simulink model "test_pkt_reorder"  (Simulink 6.2)
settings: Solver=ode45  StartTime=0.0  StopTime=200000  RelTol=1e-3
libraries: xbsIndex_r3 x556, casper_library x22, xps_library x21, simulink x1
(part 2 of 3)

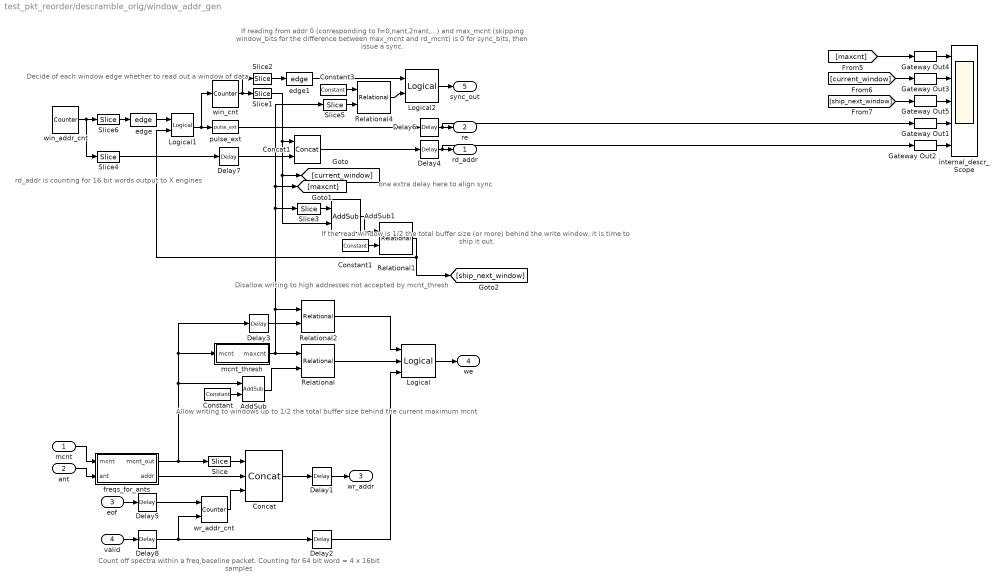
== system test_pkt_reorder/descramble_orig/window_addr_gen ==
  note: one extra delay
      | here to align sync
  note: If reading from addr 0 (corresponding to f=0,nant,2nant,...)
      | and max_mcnt (skipping window_bits for the difference
      | between max_mcnt and rd_mcnt) is 0 for sync_bits, then
      | issue a sync.
  note: Allow writing to windows
      | up to 1/2 the total buffer size
      |  behind the current maximum mcnt
  note: Count off spectra
      | within a freq,baseline
      | packet.  Counting for
      | 64 bit word = 4 x 16bit samples
  note: Decide of each window
      | edge whether to read
      | out a window of data
  note: If the read window is 1/2
      | the total buffer size (or more)
      | behind the write window,
      | it is time to ship it out.
  note: rd_addr is counting for
      | 16 bit words output to
      | X engines
  note: Disallow writing to high addresses
      | not accepted by mcnt_thresh
  mcnt : Inport  Port=1  LatchInput=off
  ant : Inport  Port=2  LatchInput=off
  eof : Inport  Port=3  LatchInput=off
  valid : Inport  Port=4  LatchInput=off
  AddSub : xbsIndex_r3/AddSub  mode=Addition  precision=User Defined  arith_type=Unsigned  n_bits=48 - ant_bits  bin_pt=0  quantization=Truncate  overflow=Wrap  latency=2  explicit_period=off  period=1  use_carryin=off  use_carryout=off  en=off  dbl_ovrd=off  show_param=off  use_core=on  pipeline=off  use_rpm=on  gen_core=off
      settings: xl_area=[0, 0, 0, 0, 0, 0, 0]
  AddSub1 : xbsIndex_r3/AddSub  mode=Subtraction  precision=User Defined  arith_type=Unsigned  n_bits=window_bits  bin_pt=0  quantization=Truncate  overflow=Wrap  latency=2  explicit_period=off  period=1  use_carryin=off  use_carryout=off  en=off  dbl_ovrd=off  show_param=off  use_core=on  pipeline=off  use_rpm=on  gen_core=off
      settings: xl_area=[0, 0, 0, 0, 0, 0, 0]
  Concat : xbsIndex_r3/Concat  num_inputs=3  explicit_period=off  period=1  dbl_ovrd=off
  Concat1 : xbsIndex_r3/Concat  num_inputs=2  explicit_period=off  period=1  dbl_ovrd=off
  Constant : xbsIndex_r3/Constant  const=2^(window_bits - 1)  equ=P=C  arith_type=Unsigned  n_bits=48 - ant_bits  bin_pt=0  opselect=C  inp2=PCIN>>17  opr=+  inp1=P  carry=CIN  iostate=0  explicit_period=on  period=1  dbl_ovrd=off
  Constant1 : xbsIndex_r3/Constant  const=2^(window_bits - 1)  equ=P=C  arith_type=Unsigned  n_bits=window_bits  bin_pt=0  opselect=C  inp2=PCIN>>17  opr=+  inp1=P  carry=CIN  iostate=0  explicit_period=on  period=1  dbl_ovrd=off
  Constant3 : xbsIndex_r3/Constant  const=0  equ=P=C  arith_type=Unsigned  n_bits=sync_bits - x_int_bits - ant_bits - window_bits  bin_pt=0  opselect=C  inp2=PCIN>>17  opr=+  inp1=P  carry=CIN  iostate=0  explicit_period=on  period=1  dbl_ovrd=off
  Delay1 : xbsIndex_r3/Delay  latency=3  reg_retiming=off  explicit_period=off  period=1  en=off  accept_only_valid=off  init_zero=on  dbl_ovrd=off  show_param=off
      settings: xl_area=[0, 0, 0, 0, 0, 0, 0]
  Delay2 : xbsIndex_r3/Delay  latency=3  reg_retiming=off  explicit_period=off  period=1  en=off  accept_only_valid=off  init_zero=on  dbl_ovrd=off  show_param=off
      settings: xl_area=[0, 0, 0, 0, 0, 0, 0]
  Delay3 : xbsIndex_r3/Delay  latency=2  reg_retiming=off  explicit_period=off  period=1  en=off  accept_only_valid=off  init_zero=on  dbl_ovrd=off  show_param=off
      settings: xl_area=[0, 0, 0, 0, 0, 0, 0]
  Delay{4..8} (5 alike) : xbsIndex_r3/Delay  latency=1  reg_retiming=off  explicit_period=off  period=1  en=off  accept_only_valid=off  init_zero=on  dbl_ovrd=off  show_param=off
      settings: xl_area=[0, 0, 0, 0, 0, 0, 0]
  Gateway Out{1..5} (5 alike) : xbsIndex_r3/Gateway Out  output_type=Double  nbits=8  bin_pt=6  arith_type=Boolean  quantization=Truncate  overflow=Wrap  hdl_port=off  timing_constraint=None  locs_specified=off  LOCs={}  needs_fixed_name=off  show_param=off
      settings: xl_area=[0, 0, 0, 0, 0, 0, 0]
  Logical : xbsIndex_r3/Logical  logical_function=AND  inputs=3  precision=Full  arith_type=Unsigned  n_bits=8  bin_pt=2  align_bp=on  latency=0  explicit_period=off  period=1  en=off  dbl_ovrd=off  show_param=off
      settings: xl_area=[0, 0, 0, 0, 0, 0, 0]
  Logical1 : xbsIndex_r3/Logical  logical_function=AND  inputs=2  precision=Full  arith_type=Unsigned  n_bits=8  bin_pt=2  align_bp=on  latency=0  explicit_period=off  period=1  en=off  dbl_ovrd=off  show_param=off
      settings: xl_area=[0, 0, 0, 0, 0, 0, 0]
  Logical2 : xbsIndex_r3/Logical  logical_function=AND  inputs=2  precision=Full  arith_type=Unsigned  n_bits=8  bin_pt=2  align_bp=on  latency=0  explicit_period=off  period=1  en=off  dbl_ovrd=off  show_param=off
      settings: xl_area=[0, 0, 0, 0, 0, 0, 0]
  Relational : xbsIndex_r3/Relational  mode=a<b  latency=1  explicit_period=off  period=1  en=off  dbl_ovrd=off  show_param=off
      settings: xl_area=[0, 0, 0, 0, 0, 0, 0]
  Relational1 : xbsIndex_r3/Relational  mode=a>=b  latency=1  explicit_period=on  period=1  en=off  dbl_ovrd=off  show_param=off
      settings: xl_area=[0, 0, 0, 0, 0, 0, 0]
  Relational2 : xbsIndex_r3/Relational  mode=a>=b  latency=1  explicit_period=off  period=1  en=off  dbl_ovrd=off  show_param=off
      settings: xl_area=[0, 0, 0, 0, 0, 0, 0]
  Relational4 : xbsIndex_r3/Relational  mode=a=b  latency=1  explicit_period=off  period=1  en=off  dbl_ovrd=off  show_param=off
      settings: xl_area=[0, 0, 0, 0, 0, 0, 0]
  Slice : xbsIndex_r3/Slice  mode=Lower Bit Location + Width  nbits=window_bits  bit1=0  base1=MSB of Input  bit0=0  base0=LSB of Input  boolean_output=off  explicit_period=off  period=1  dbl_ovrd=off
  Slice1 : xbsIndex_r3/Slice  mode=Lower Bit Location + Width  nbits=window_bits  bit1=0  base1=MSB of Input  bit0=0  base0=LSB of Input  boolean_output=off  explicit_period=off  period=1  dbl_ovrd=off
  Slice2 : xbsIndex_r3/Slice  mode=Upper Bit Location + Width  nbits=1  bit1=0  base1=MSB of Input  bit0=0  base0=LSB of Input  boolean_output=on  explicit_period=off  period=1  dbl_ovrd=off
  Slice3 : xbsIndex_r3/Slice  mode=Lower Bit Location + Width  nbits=window_bits  bit1=0  base1=MSB of Input  bit0=0  base0=LSB of Input  boolean_output=off  explicit_period=off  period=1  dbl_ovrd=off
  Slice4 : xbsIndex_r3/Slice  mode=Lower Bit Location + Width  nbits=x_int_bits + ant_bits  bit1=0  base1=MSB of Input  bit0=0  base0=LSB of Input  boolean_output=off  explicit_period=off  period=1  dbl_ovrd=off
  Slice5 : xbsIndex_r3/Slice  mode=Two Bit Locations  nbits=window_bits  bit1=sync_bits - x_int_bits - ant_bits - 1  base1=LSB of Input  bit0=window_bits  base0=LSB of Input  boolean_output=off  explicit_period=off  period=1  dbl_ovrd=off
  Slice6 : xbsIndex_r3/Slice  mode=Upper Bit Location + Width  nbits=1  bit1=0  base1=MSB of Input  bit0=0  base0=LSB of Input  boolean_output=on  explicit_period=off  period=1  dbl_ovrd=off
  edge : casper_library/Misc/edge
  edge1 : casper_library/Misc/edge
  freqs_for_ants : Subsystem
  internal_descr_Scope : Scope  NumInputPorts=5
      settings: TimeRange=1  YMin=-1~-1~0.95~-5~-5  YMax=1~1~1.05~5~5  SaveName=ScopeData4
  mcnt_thresh : Subsystem
  pulse_ext : casper_library/Misc/pulse_ext  pulse_len=2^(x_int_bits + ant_bits)
  win_addr_cnt : xbsIndex_r3/Counter  cnt_type=Free Running  n_bits=x_int_bits + ant_bits + 1  bin_pt=0  arith_type=Unsigned  start_count=0  cnt_to=Inf  cnt_by_val=1  operation=Up  explicit_period=off  period=1  load_pin=off  rst=off  en=off  dbl_ovrd=off  show_param=off  use_rpm=on  gen_core=off
      settings: xl_area=[0, 0, 0, 0, 0, 0, 0]
  win_cnt : xbsIndex_r3/Counter  cnt_type=Free Running  n_bits=window_bits + 1  bin_pt=0  arith_type=Unsigned  start_count=0  cnt_to=Inf  cnt_by_val=1  operation=Up  explicit_period=off  period=1  load_pin=off  rst=off  en=on  dbl_ovrd=off  show_param=off  use_rpm=on  gen_core=off
      settings: xl_area=[0, 0, 0, 0, 0, 0, 0]
  wr_addr_cnt : xbsIndex_r3/Counter  cnt_type=Free Running  n_bits=x_int_bits - 2  bin_pt=0  arith_type=Unsigned  start_count=0  cnt_to=Inf  cnt_by_val=1  operation=Up  explicit_period=off  period=1  load_pin=off  rst=on  en=on  dbl_ovrd=off  show_param=off  use_rpm=on  gen_core=off
      settings: xl_area=[0, 0, 0, 0, 0, 0, 0]
  rd_addr : Outport
  re : Outport  Port=2
  wr_addr : Outport  Port=3
  we : Outport  Port=4
  sync_out : Outport  Port=5
  wires:
  pulse_ext/1 -> Delay6/1
  Concat1/1 -> Delay4/1
  Delay7/1 -> Concat1/2
  Slice2/1 -> edge1/1
  Slice1/1 -> Concat1/1, AddSub1/2, [current_window]
  Slice4/1 -> Delay7/1
  freqs_for_ants/1(mcnt_out) -> Delay3/1, mcnt_thresh/1(mcnt), AddSub/1, Slice/1
  edge/1 -> Logical1/1
  Slice6/1 -> edge/1
  win_addr_cnt/1 -> Slice4/1, Slice6/1
  Delay6/1 -> re/1, Gateway Out1/1
  Delay4/1 -> rd_addr/1, Gateway Out2/1
  Relational1/1 -> Logical1/2, [ship_next_window]
  Logical2/1 -> sync_out/1
  Relational4/1 -> Logical2/2
  Slice5/1 -> Relational4/2
  Constant3/1 -> Relational4/1
  edge1/1 -> Logical2/1
  Delay3/1 -> Relational2/2
  Relational2/1 -> Logical/1
  mcnt_thresh/1(maxcnt) -> Relational2/1, Slice3/1, Slice5/1, [maxcnt], Relational/1
  Constant/1 -> AddSub/2
  mcnt/1 -> freqs_for_ants/1(mcnt)
  AddSub/1 -> Relational/2
  Slice/1 -> Concat/1
  freqs_for_ants/2(addr) -> Concat/2
  Concat/1 -> Delay1/1
  Delay1/1 -> wr_addr/1
  ant/1 -> freqs_for_ants/2(ant)
  wr_addr_cnt/1 -> Concat/3
  valid/1 -> Delay8/1
  eof/1 -> Delay5/1
  Relational/1 -> Logical/2
  Logical/1 -> we/1
  Delay2/1 -> Logical/3
  Logical1/1 -> win_cnt/1, pulse_ext/1
  Slice3/1 -> AddSub1/1
  win_cnt/1 -> Slice2/1, Slice1/1
  AddSub1/1 -> Relational1/1
  Constant1/1 -> Relational1/2
  Delay5/1 -> wr_addr_cnt/1
  Delay8/1 -> wr_addr_cnt/2, Delay2/1
  Gateway Out3/1 -> internal_descr_Scope/2
  Gateway Out4/1 -> internal_descr_Scope/1
  Gateway Out5/1 -> internal_descr_Scope/3
  Gateway Out1/1 -> internal_descr_Scope/4
  Gateway Out2/1 -> internal_descr_Scope/5
  [maxcnt] -> Gateway Out4/1
  [current_window] -> Gateway Out3/1
  [ship_next_window] -> Gateway Out5/1

== system test_pkt_reorder/descramble_window0/deflagger ==
  din : Inport  Port=1  LatchInput=off
  Slice1 : xbsIndex_r3/Slice  mode=Lower Bit Location + Width  nbits=16  bit1=0  base1=MSB of Input  bit0=0  base0=LSB of Input  boolean_output=off  explicit_period=off  period=1  dbl_ovrd=off
  Slice2 : xbsIndex_r3/Slice  mode=Upper Bit Location + Width  nbits=1  bit1=-1  base1=MSB of Input  bit0=0  base0=LSB of Input  boolean_output=on  explicit_period=off  period=1  dbl_ovrd=off
  Slice3 : xbsIndex_r3/Slice  mode=Upper Bit Location + Width  nbits=1  bit1=0  base1=MSB of Input  bit0=0  base0=LSB of Input  boolean_output=on  explicit_period=off  period=1  dbl_ovrd=off
  dout : Outport
  flag : Outport  Port=2
  rcvd : Outport  Port=3
  wires:
  Slice1/1 -> dout/1
  Slice3/1 -> rcvd/1
  Slice2/1 -> flag/1
  din/1 -> Slice3/1, Slice2/1, Slice1/1

== system test_pkt_reorder/descramble_window0/flagger ==
  flag : Inport  Port=1  LatchInput=off
  din : Inport  Port=2  LatchInput=off
  Concat : xbsIndex_r3/Concat  num_inputs=12  explicit_period=off  period=1  dbl_ovrd=off
  Constant{1..4} (4 alike) : xbsIndex_r3/Constant  const=1  equ=P=C  arith_type=Unsigned  n_bits=1  bin_pt=0  opselect=C  inp2=PCIN>>17  opr=+  inp1=P  carry=CIN  iostate=0  explicit_period=on  period=1  dbl_ovrd=off
  Slice1 : xbsIndex_r3/Slice  mode=Lower Bit Location + Width  nbits=16  bit1=0  base1=MSB of Input  bit0=0  base0=LSB of Input  boolean_output=off  explicit_period=off  period=1  dbl_ovrd=off
  Slice2 : xbsIndex_r3/Slice  mode=Lower Bit Location + Width  nbits=16  bit1=0  base1=MSB of Input  bit0=16  base0=LSB of Input  boolean_output=off  explicit_period=off  period=1  dbl_ovrd=off
  Slice3 : xbsIndex_r3/Slice  mode=Lower Bit Location + Width  nbits=16  bit1=0  base1=MSB of Input  bit0=32  base0=LSB of Input  boolean_output=off  explicit_period=off  period=1  dbl_ovrd=off
  Slice4 : xbsIndex_r3/Slice  mode=Lower Bit Location + Width  nbits=16  bit1=0  base1=MSB of Input  bit0=48  base0=LSB of Input  boolean_output=off  explicit_period=off  period=1  dbl_ovrd=off
  dout : Outport
  wires:
  Concat/1 -> dout/1
  din/1 -> Slice4/1, Slice3/1, Slice2/1, Slice1/1
  flag/1 -> Concat/11, Concat/8, Concat/5, Concat/2
  Slice4/1 -> Concat/12
  Slice3/1 -> Concat/9
  Slice2/1 -> Concat/6
  Slice1/1 -> Concat/3
  Constant1/1 -> Concat/10
  Constant2/1 -> Concat/7
  Constant3/1 -> Concat/4
  Constant4/1 -> Concat/1

== system test_pkt_reorder/descramble_window0/window_addr_gen ==
  note: Allow writing to windows
      | up to 1/2 the total buffer size
      |  behind the current maximum mcnt
  note: Count off spectra
      | within a freq,baseline
      | packet.  Counting for
      | 64 bit word = 4 x 16bit samples
  note: Disallow writing to high addresses
      | not accepted by mcnt_thresh
  note: This block ignores
      | MCNTs destined for other X engines
  mcnt : Inport  Port=1  LatchInput=off
  ant : Inport  Port=2  LatchInput=off
  eof : Inport  Port=3  LatchInput=off
  valid : Inport  Port=4  LatchInput=off
  AddSub : xbsIndex_r3/AddSub  mode=Addition  precision=User Defined  arith_type=Unsigned  n_bits=48 - ant_bits  bin_pt=0  quantization=Truncate  overflow=Wrap  latency=2  explicit_period=off  period=1  use_carryin=off  use_carryout=off  en=off  dbl_ovrd=off  show_param=off  use_core=on  pipeline=off  use_rpm=on  gen_core=off
      settings: xl_area=[0, 0, 0, 0, 0, 0, 0]
  Concat : xbsIndex_r3/Concat  num_inputs=3  explicit_period=off  period=1  dbl_ovrd=off
  Constant : xbsIndex_r3/Constant  const=2^(window_bits - 1)  equ=P=C  arith_type=Unsigned  n_bits=48 - ant_bits  bin_pt=0  opselect=C  inp2=PCIN>>17  opr=+  inp1=P  carry=CIN  iostate=0  explicit_period=on  period=1  dbl_ovrd=off
  Delay1 : xbsIndex_r3/Delay  latency=3  reg_retiming=off  explicit_period=off  period=1  en=off  accept_only_valid=off  init_zero=on  dbl_ovrd=off  show_param=off
      settings: xl_area=[0, 0, 0, 0, 0, 0, 0]
  Delay2 : xbsIndex_r3/Delay  latency=3  reg_retiming=off  explicit_period=off  period=1  en=off  accept_only_valid=off  init_zero=on  dbl_ovrd=off  show_param=off
      settings: xl_area=[0, 0, 0, 0, 0, 0, 0]
  Delay3 : xbsIndex_r3/Delay  latency=2  reg_retiming=off  explicit_period=off  period=1  en=off  accept_only_valid=off  init_zero=on  dbl_ovrd=off  show_param=off
      settings: xl_area=[0, 0, 0, 0, 0, 0, 0]
  Delay{4..6,8} (4 alike) : xbsIndex_r3/Delay  latency=1  reg_retiming=on  explicit_period=off  period=1  en=off  accept_only_valid=off  init_zero=on  dbl_ovrd=off  show_param=off
      settings: xl_area=[0, 0, 0, 0, 0, 0, 0]
  Logical : xbsIndex_r3/Logical  logical_function=AND  inputs=3  precision=Full  arith_type=Unsigned  n_bits=8  bin_pt=2  align_bp=on  latency=0  explicit_period=off  period=1  en=off  dbl_ovrd=off  show_param=off
      settings: xl_area=[0, 0, 0, 0, 0, 0, 0]
  Logical1 : xbsIndex_r3/Logical  logical_function=AND  inputs=2  precision=Full  arith_type=Unsigned  n_bits=8  bin_pt=2  align_bp=on  latency=0  explicit_period=off  period=1  en=off  dbl_ovrd=off  show_param=off
      settings: xl_area=[0, 0, 0, 0, 0, 0, 0]
  Relational : xbsIndex_r3/Relational  mode=a<b  latency=1  explicit_period=off  period=1  en=off  dbl_ovrd=off  show_param=off
      settings: xl_area=[0, 0, 0, 0, 0, 0, 0]
  Relational2 : xbsIndex_r3/Relational  mode=a>=b  latency=1  explicit_period=off  period=1  en=off  dbl_ovrd=off  show_param=off
      settings: xl_area=[0, 0, 0, 0, 0, 0, 0]
  Slice : xbsIndex_r3/Slice  mode=Lower Bit Location + Width  nbits=window_bits  bit1=0  base1=MSB of Input  bit0=0  base0=LSB of Input  boolean_output=off  explicit_period=off  period=1  dbl_ovrd=off
  Slice1 : xbsIndex_r3/Slice  mode=Lower Bit Location + Width  nbits=ant_bits  bit1=0  base1=MSB of Input  bit0=0  base0=LSB of Input  boolean_output=off  explicit_period=off  period=1  dbl_ovrd=off
  Slice14 : xbsIndex_r3/Slice  mode=Two Bit Locations  nbits=ant_bits  bit1=0  base1=MSB of Input  bit0=xeng_bits  base0=LSB of Input  boolean_output=off  explicit_period=off  period=1  dbl_ovrd=off
  mcnt_thresh : Subsystem
  output_control : Subsystem
  wr_addr_cnt : xbsIndex_r3/Counter  cnt_type=Free Running  n_bits=x_int_bits - 2  bin_pt=0  arith_type=Unsigned  start_count=0  cnt_to=Inf  cnt_by_val=1  operation=Up  explicit_period=off  period=1  load_pin=off  rst=on  en=on  dbl_ovrd=off  show_param=off  use_rpm=on  gen_core=off
      settings: xl_area=[0, 0, 0, 0, 0, 0, 0]
  rd_addr : Outport
  re : Outport  Port=2
  wr_addr : Outport  Port=3
  we : Outport  Port=4
  sync_out : Outport  Port=5
  maxcnt : Outport  Port=6
  wires:
  Slice14/1 -> Delay5/1
  output_control/2(rd_en) -> re/1
  output_control/3(rd_addr) -> rd_addr/1
  output_control/1(gen_sync) -> sync_out/1
  Delay3/1 -> Relational2/2
  Relational2/1 -> Logical/1
  mcnt_thresh/1(maxcnt) -> Relational2/1, maxcnt/1, output_control/1(maxcnt), Relational/1
  Constant/1 -> AddSub/2
  AddSub/1 -> Relational/2
  Slice/1 -> Concat/1
  Slice1/1 -> Delay6/1
  Concat/1 -> Delay1/1
  Delay1/1 -> wr_addr/1
  wr_addr_cnt/1 -> Concat/3
  valid/1 -> Delay8/1, Logical1/2
  Relational/1 -> Logical/2
  Logical/1 -> we/1
  Delay2/1 -> Logical/3
  Delay4/1 -> wr_addr_cnt/1
  Delay8/1 -> wr_addr_cnt/2, Delay2/1
  mcnt/1 -> Slice14/1
  ant/1 -> Slice1/1
  Logical1/1 -> Delay4/1
  eof/1 -> Logical1/1
  Delay5/1 -> Delay3/1, mcnt_thresh/1(mcnt), AddSub/1, Slice/1
  Delay6/1 -> Concat/2

== system test_pkt_reorder/descramble_window1/deflagger ==
  din : Inport  Port=1  LatchInput=off
  Slice1 : xbsIndex_r3/Slice  mode=Lower Bit Location + Width  nbits=16  bit1=0  base1=MSB of Input  bit0=0  base0=LSB of Input  boolean_output=off  explicit_period=off  period=1  dbl_ovrd=off
  Slice2 : xbsIndex_r3/Slice  mode=Upper Bit Location + Width  nbits=1  bit1=-1  base1=MSB of Input  bit0=0  base0=LSB of Input  boolean_output=on  explicit_period=off  period=1  dbl_ovrd=off
  Slice3 : xbsIndex_r3/Slice  mode=Upper Bit Location + Width  nbits=1  bit1=0  base1=MSB of Input  bit0=0  base0=LSB of Input  boolean_output=on  explicit_period=off  period=1  dbl_ovrd=off
  dout : Outport
  flag : Outport  Port=2
  rcvd : Outport  Port=3
  wires:
  Slice1/1 -> dout/1
  Slice3/1 -> rcvd/1
  Slice2/1 -> flag/1
  din/1 -> Slice3/1, Slice2/1, Slice1/1

== system test_pkt_reorder/descramble_window1/flagger ==
  flag : Inport  Port=1  LatchInput=off
  din : Inport  Port=2  LatchInput=off
  Concat : xbsIndex_r3/Concat  num_inputs=12  explicit_period=off  period=1  dbl_ovrd=off
  Constant{1..4} (4 alike) : xbsIndex_r3/Constant  const=1  equ=P=C  arith_type=Unsigned  n_bits=1  bin_pt=0  opselect=C  inp2=PCIN>>17  opr=+  inp1=P  carry=CIN  iostate=0  explicit_period=on  period=1  dbl_ovrd=off
  Slice1 : xbsIndex_r3/Slice  mode=Lower Bit Location + Width  nbits=16  bit1=0  base1=MSB of Input  bit0=0  base0=LSB of Input  boolean_output=off  explicit_period=off  period=1  dbl_ovrd=off
  Slice2 : xbsIndex_r3/Slice  mode=Lower Bit Location + Width  nbits=16  bit1=0  base1=MSB of Input  bit0=16  base0=LSB of Input  boolean_output=off  explicit_period=off  period=1  dbl_ovrd=off
  Slice3 : xbsIndex_r3/Slice  mode=Lower Bit Location + Width  nbits=16  bit1=0  base1=MSB of Input  bit0=32  base0=LSB of Input  boolean_output=off  explicit_period=off  period=1  dbl_ovrd=off
  Slice4 : xbsIndex_r3/Slice  mode=Lower Bit Location + Width  nbits=16  bit1=0  base1=MSB of Input  bit0=48  base0=LSB of Input  boolean_output=off  explicit_period=off  period=1  dbl_ovrd=off
  dout : Outport
  wires:
  Concat/1 -> dout/1
  din/1 -> Slice4/1, Slice3/1, Slice2/1, Slice1/1
  flag/1 -> Concat/11, Concat/8, Concat/5, Concat/2
  Slice4/1 -> Concat/12
  Slice3/1 -> Concat/9
  Slice2/1 -> Concat/6
  Slice1/1 -> Concat/3
  Constant1/1 -> Concat/10
  Constant2/1 -> Concat/7
  Constant3/1 -> Concat/4
  Constant4/1 -> Concat/1

== system test_pkt_reorder/descramble_window1/window_addr_gen ==
  note: Allow writing to windows
      | up to 1/2 the total buffer size
      |  behind the current maximum mcnt
  note: Count off spectra
      | within a freq,baseline
      | packet.  Counting for
      | 64 bit word = 4 x 16bit samples
  note: Disallow writing to high addresses
      | not accepted by mcnt_thresh
  note: This block ignores
      | MCNTs destined for other X engines
  mcnt : Inport  Port=1  LatchInput=off
  ant : Inport  Port=2  LatchInput=off
  eof : Inport  Port=3  LatchInput=off
  valid : Inport  Port=4  LatchInput=off
  AddSub : xbsIndex_r3/AddSub  mode=Addition  precision=User Defined  arith_type=Unsigned  n_bits=48 - ant_bits  bin_pt=0  quantization=Truncate  overflow=Wrap  latency=2  explicit_period=off  period=1  use_carryin=off  use_carryout=off  en=off  dbl_ovrd=off  show_param=off  use_core=on  pipeline=off  use_rpm=on  gen_core=off
      settings: xl_area=[0, 0, 0, 0, 0, 0, 0]
  Concat : xbsIndex_r3/Concat  num_inputs=3  explicit_period=off  period=1  dbl_ovrd=off
  Constant : xbsIndex_r3/Constant  const=2^(window_bits - 1)  equ=P=C  arith_type=Unsigned  n_bits=48 - ant_bits  bin_pt=0  opselect=C  inp2=PCIN>>17  opr=+  inp1=P  carry=CIN  iostate=0  explicit_period=on  period=1  dbl_ovrd=off
  Delay1 : xbsIndex_r3/Delay  latency=3  reg_retiming=off  explicit_period=off  period=1  en=off  accept_only_valid=off  init_zero=on  dbl_ovrd=off  show_param=off
      settings: xl_area=[0, 0, 0, 0, 0, 0, 0]
  Delay2 : xbsIndex_r3/Delay  latency=3  reg_retiming=off  explicit_period=off  period=1  en=off  accept_only_valid=off  init_zero=on  dbl_ovrd=off  show_param=off
      settings: xl_area=[0, 0, 0, 0, 0, 0, 0]
  Delay3 : xbsIndex_r3/Delay  latency=2  reg_retiming=off  explicit_period=off  period=1  en=off  accept_only_valid=off  init_zero=on  dbl_ovrd=off  show_param=off
      settings: xl_area=[0, 0, 0, 0, 0, 0, 0]
  Delay4 : xbsIndex_r3/Delay  latency=1  reg_retiming=on  explicit_period=off  period=1  en=off  accept_only_valid=off  init_zero=on  dbl_ovrd=off  show_param=off
      settings: xl_area=[0, 0, 0, 0, 0, 0, 0]
  Delay8 : xbsIndex_r3/Delay  latency=1  reg_retiming=on  explicit_period=off  period=1  en=off  accept_only_valid=off  init_zero=on  dbl_ovrd=off  show_param=off
      settings: xl_area=[0, 0, 0, 0, 0, 0, 0]
  Logical : xbsIndex_r3/Logical  logical_function=AND  inputs=3  precision=Full  arith_type=Unsigned  n_bits=8  bin_pt=2  align_bp=on  latency=0  explicit_period=off  period=1  en=off  dbl_ovrd=off  show_param=off
      settings: xl_area=[0, 0, 0, 0, 0, 0, 0]
  Logical1 : xbsIndex_r3/Logical  logical_function=AND  inputs=2  precision=Full  arith_type=Unsigned  n_bits=8  bin_pt=2  align_bp=on  latency=0  explicit_period=off  period=1  en=off  dbl_ovrd=off  show_param=off
      settings: xl_area=[0, 0, 0, 0, 0, 0, 0]
  Relational : xbsIndex_r3/Relational  mode=a<b  latency=1  explicit_period=off  period=1  en=off  dbl_ovrd=off  show_param=off
      settings: xl_area=[0, 0, 0, 0, 0, 0, 0]
  Relational2 : xbsIndex_r3/Relational  mode=a>=b  latency=1  explicit_period=off  period=1  en=off  dbl_ovrd=off  show_param=off
      settings: xl_area=[0, 0, 0, 0, 0, 0, 0]
  Slice : xbsIndex_r3/Slice  mode=Lower Bit Location + Width  nbits=window_bits  bit1=0  base1=MSB of Input  bit0=0  base0=LSB of Input  boolean_output=off  explicit_period=off  period=1  dbl_ovrd=off
  Slice1 : xbsIndex_r3/Slice  mode=Lower Bit Location + Width  nbits=ant_bits  bit1=0  base1=MSB of Input  bit0=0  base0=LSB of Input  boolean_output=off  explicit_period=off  period=1  dbl_ovrd=off
  Slice14 : xbsIndex_r3/Slice  mode=Two Bit Locations  nbits=ant_bits  bit1=0  base1=MSB of Input  bit0=xeng_bits  base0=LSB of Input  boolean_output=off  explicit_period=off  period=1  dbl_ovrd=off
  mcnt_thresh : Subsystem
  output_control : Subsystem
  wr_addr_cnt : xbsIndex_r3/Counter  cnt_type=Free Running  n_bits=x_int_bits - 2  bin_pt=0  arith_type=Unsigned  start_count=0  cnt_to=Inf  cnt_by_val=1  operation=Up  explicit_period=off  period=1  load_pin=off  rst=on  en=on  dbl_ovrd=off  show_param=off  use_rpm=on  gen_core=off
      settings: xl_area=[0, 0, 0, 0, 0, 0, 0]
  rd_addr : Outport
  re : Outport  Port=2
  wr_addr : Outport  Port=3
  we : Outport  Port=4
  sync_out : Outport  Port=5
  maxcnt : Outport  Port=6
  wires:
  Slice14/1 -> Delay3/1, mcnt_thresh/1(mcnt), AddSub/1, Slice/1
  output_control/2(rd_en) -> re/1
  output_control/3(rd_addr) -> rd_addr/1
  output_control/1(gen_sync) -> sync_out/1
  Delay3/1 -> Relational2/2
  Relational2/1 -> Logical/1
  mcnt_thresh/1(maxcnt) -> Relational2/1, maxcnt/1, output_control/1(maxcnt), Relational/1
  Constant/1 -> AddSub/2
  AddSub/1 -> Relational/2
  Slice/1 -> Concat/1
  Slice1/1 -> Concat/2
  Concat/1 -> Delay1/1
  Delay1/1 -> wr_addr/1
  wr_addr_cnt/1 -> Concat/3
  valid/1 -> Delay8/1, Logical1/2
  Relational/1 -> Logical/2
  Logical/1 -> we/1
  Delay2/1 -> Logical/3
  Delay4/1 -> wr_addr_cnt/1
  Delay8/1 -> wr_addr_cnt/2, Delay2/1
  mcnt/1 -> Slice14/1
  ant/1 -> Slice1/1
  Logical1/1 -> Delay4/1
  eof/1 -> Logical1/1

== system test_pkt_reorder/pkt_reord0/deflagger ==
  din : Inport  Port=1  LatchInput=off
  Slice1 : xbsIndex_r3/Slice  mode=Lower Bit Location + Width  nbits=16  bit1=0  base1=MSB of Input  bit0=0  base0=LSB of Input  boolean_output=off  explicit_period=off  period=1  dbl_ovrd=off
  Slice2 : xbsIndex_r3/Slice  mode=Upper Bit Location + Width  nbits=1  bit1=-1  base1=MSB of Input  bit0=0  base0=LSB of Input  boolean_output=on  explicit_period=off  period=1  dbl_ovrd=off
  Slice3 : xbsIndex_r3/Slice  mode=Upper Bit Location + Width  nbits=1  bit1=0  base1=MSB of Input  bit0=0  base0=LSB of Input  boolean_output=on  explicit_period=off  period=1  dbl_ovrd=off
  dout : Outport
  flag : Outport  Port=2
  rcvd : Outport  Port=3
  wires:
  Slice1/1 -> dout/1
  Slice3/1 -> rcvd/1
  Slice2/1 -> flag/1
  din/1 -> Slice3/1, Slice2/1, Slice1/1

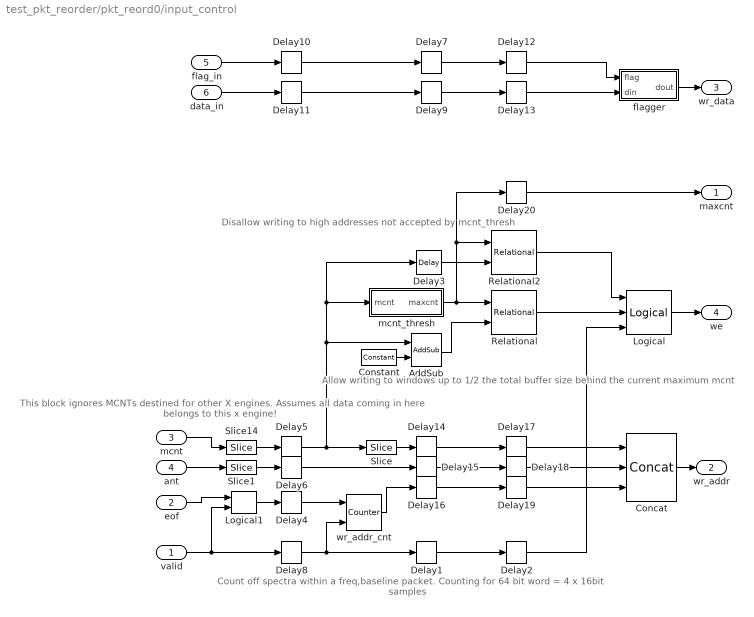
== system test_pkt_reorder/pkt_reord0/input_control ==
  note: Allow writing to windows
      | up to 1/2 the total buffer size
      |  behind the current maximum mcnt
  note: Count off spectra
      | within a freq,baseline
      | packet.  Counting for
      | 64 bit word = 4 x 16bit samples
  note: Disallow writing to high addresses
      | not accepted by mcnt_thresh
  note: This block ignores
      | MCNTs destined for other X engines.
      | Assumes all data coming in here
      | belongs to this x engine!
  valid : Inport  Port=1  LatchInput=off
  eof : Inport  Port=2  LatchInput=off
  mcnt : Inport  Port=3  LatchInput=off
  ant : Inport  Port=4  LatchInput=off
  flag_in : Inport  Port=5  LatchInput=off
  data_in : Inport  Port=6  LatchInput=off
  AddSub : xbsIndex_r3/AddSub  mode=Addition  precision=User Defined  arith_type=Unsigned  n_bits=48 - ant_bits  bin_pt=0  quantization=Truncate  overflow=Wrap  latency=2  explicit_period=off  period=1  use_carryin=off  use_carryout=off  en=off  dbl_ovrd=off  show_param=off  use_core=on  pipeline=off  use_rpm=on  gen_core=off
      settings: xl_area=[0, 0, 0, 0, 0, 0, 0]
  Concat : xbsIndex_r3/Concat  num_inputs=3  explicit_period=off  period=1  dbl_ovrd=off
  Constant : xbsIndex_r3/Constant  const=2^(window_bits - 1)  equ=P=C  arith_type=Unsigned  n_bits=48 - ant_bits  bin_pt=0  opselect=C  inp2=PCIN>>17  opr=+  inp1=P  carry=CIN  iostate=0  explicit_period=on  period=1  dbl_ovrd=off
  Delay{1,7,9,14..16} (6 alike) : xbsIndex_r3/Delay  latency=2  reg_retiming=on  explicit_period=off  period=1  en=off  accept_only_valid=off  init_zero=on  dbl_ovrd=off  show_param=off
      settings: xl_area=[0, 0, 0, 0, 0, 0, 0]
  Delay{2,4..6,8,10..13,17..20} (13 alike) : xbsIndex_r3/Delay  latency=1  reg_retiming=on  explicit_period=off  period=1  en=off  accept_only_valid=off  init_zero=on  dbl_ovrd=off  show_param=off
      settings: xl_area=[0, 0, 0, 0, 0, 0, 0]
  Delay3 : xbsIndex_r3/Delay  latency=2  reg_retiming=off  explicit_period=off  period=1  en=off  accept_only_valid=off  init_zero=on  dbl_ovrd=off  show_param=off
      settings: xl_area=[0, 0, 0, 0, 0, 0, 0]
  Logical : xbsIndex_r3/Logical  logical_function=AND  inputs=3  precision=Full  arith_type=Unsigned  n_bits=8  bin_pt=2  align_bp=on  latency=0  explicit_period=off  period=1  en=off  dbl_ovrd=off  show_param=off
      settings: xl_area=[0, 0, 0, 0, 0, 0, 0]
  Logical1 : xbsIndex_r3/Logical  logical_function=AND  inputs=2  precision=Full  arith_type=Unsigned  n_bits=8  bin_pt=2  align_bp=on  latency=0  explicit_period=off  period=1  en=off  dbl_ovrd=off  show_param=off
      settings: xl_area=[0, 0, 0, 0, 0, 0, 0]
  Relational : xbsIndex_r3/Relational  mode=a<b  latency=1  explicit_period=off  period=1  en=off  dbl_ovrd=off  show_param=off
      settings: xl_area=[0, 0, 0, 0, 0, 0, 0]
  Relational2 : xbsIndex_r3/Relational  mode=a>=b  latency=1  explicit_period=off  period=1  en=off  dbl_ovrd=off  show_param=off
      settings: xl_area=[0, 0, 0, 0, 0, 0, 0]
  Slice : xbsIndex_r3/Slice  mode=Lower Bit Location + Width  nbits=window_bits  bit1=0  base1=MSB of Input  bit0=0  base0=LSB of Input  boolean_output=off  explicit_period=off  period=1  dbl_ovrd=off
  Slice1 : xbsIndex_r3/Slice  mode=Lower Bit Location + Width  nbits=ant_bits  bit1=0  base1=MSB of Input  bit0=0  base0=LSB of Input  boolean_output=off  explicit_period=off  period=1  dbl_ovrd=off
  Slice14 : xbsIndex_r3/Slice  mode=Two Bit Locations  nbits=ant_bits  bit1=0  base1=MSB of Input  bit0=xeng_bits  base0=LSB of Input  boolean_output=off  explicit_period=off  period=1  dbl_ovrd=off
  flagger : Subsystem
  mcnt_thresh : Subsystem
  wr_addr_cnt : xbsIndex_r3/Counter  cnt_type=Free Running  n_bits=x_int_bits - 2  bin_pt=0  arith_type=Unsigned  start_count=0  cnt_to=Inf  cnt_by_val=1  operation=Up  explicit_period=off  period=1  load_pin=off  rst=on  en=on  dbl_ovrd=off  show_param=off  use_rpm=on  gen_core=off
      settings: xl_area=[0, 0, 0, 0, 0, 0, 0]
  maxcnt : Outport
  wr_addr : Outport  Port=2
  wr_data : Outport  Port=3
  we : Outport  Port=4
  wires:
  Slice14/1 -> Delay5/1
  Delay3/1 -> Relational2/2
  Relational2/1 -> Logical/1
  mcnt_thresh/1(maxcnt) -> Relational2/1, Delay20/1, Relational/1
  Constant/1 -> AddSub/2
  AddSub/1 -> Relational/2
  Slice/1 -> Delay14/1
  Slice1/1 -> Delay6/1
  wr_addr_cnt/1 -> Delay16/1
  valid/1 -> Delay8/1, Logical1/2
  Relational/1 -> Logical/2
  Logical/1 -> we/1
  Delay2/1 -> Logical/3
  Delay4/1 -> wr_addr_cnt/1
  Delay8/1 -> wr_addr_cnt/2, Delay1/1
  mcnt/1 -> Slice14/1
  ant/1 -> Slice1/1
  Logical1/1 -> Delay4/1
  eof/1 -> Logical1/1
  Delay5/1 -> Delay3/1, mcnt_thresh/1(mcnt), AddSub/1, Slice/1
  Delay6/1 -> Delay15/1
  Delay7/1 -> Delay12/1
  data_in/1 -> Delay11/1
  Delay9/1 -> Delay13/1
  flag_in/1 -> Delay10/1
  flagger/1(dout) -> wr_data/1
  Delay10/1 -> Delay7/1
  Delay11/1 -> Delay9/1
  Delay12/1 -> flagger/1(flag)
  Delay13/1 -> flagger/2(din)
  Concat/1 -> wr_addr/1
  Delay1/1 -> Delay2/1
  Delay16/1 -> Delay19/1
  Delay15/1 -> Delay18/1
  Delay14/1 -> Delay17/1
  Delay17/1 -> Concat/1
  Delay18/1 -> Concat/2
  Delay19/1 -> Concat/3
  Delay20/1 -> maxcnt/1

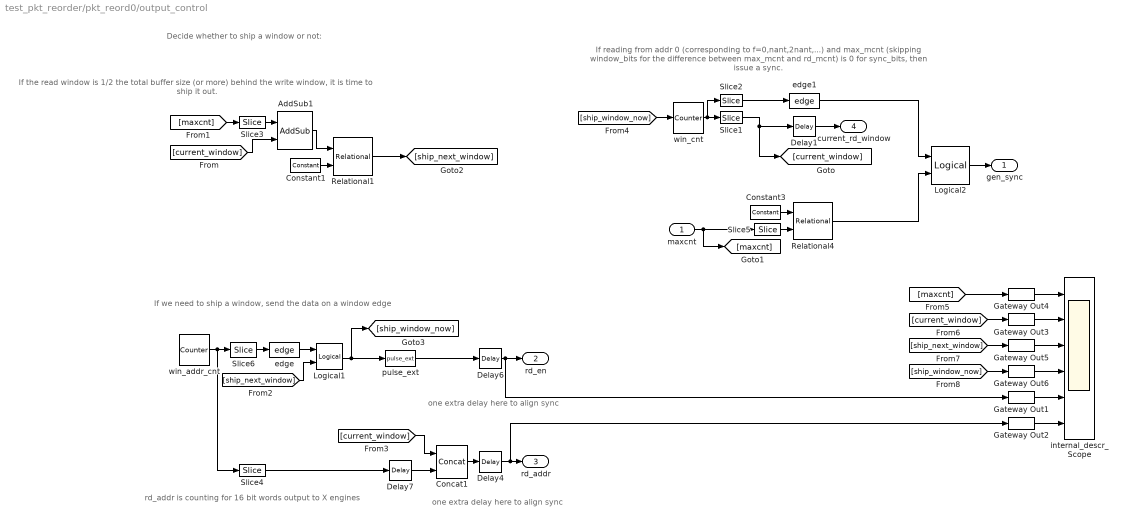
== system test_pkt_reorder/pkt_reord0/output_control ==
  note: one extra delay
      | here to align sync
  note: rd_addr is counting for
      | 16 bit words output to
      | X engines
  note: If the read window is 1/2
      | the total buffer size (or more)
      | behind the write window,
      | it is time to ship it out.
  note: one extra delay
      | here to align sync
  note: Decide whether to ship
      | a window or not:
  note: If we need to ship a window,
      | send the data on a window edge
  note: If reading from addr 0 (corresponding to f=0,nant,2nant,...)
      | and max_mcnt (skipping window_bits for the difference
      | between max_mcnt and rd_mcnt) is 0 for sync_bits, then
      | issue a sync.
  maxcnt : Inport  Port=1  LatchInput=off
  AddSub1 : xbsIndex_r3/AddSub  mode=Subtraction  precision=User Defined  arith_type=Unsigned  n_bits=window_bits  bin_pt=0  quantization=Truncate  overflow=Wrap  latency=2  explicit_period=off  period=1  use_carryin=off  use_carryout=off  en=off  dbl_ovrd=off  show_param=off  use_core=on  pipeline=off  use_rpm=on  gen_core=off
      settings: xl_area=[0, 0, 0, 0, 0, 0, 0]
  Concat1 : xbsIndex_r3/Concat  num_inputs=2  explicit_period=off  period=1  dbl_ovrd=off
  Constant1 : xbsIndex_r3/Constant  const=2^(window_bits - 1)  equ=P=C  arith_type=Unsigned  n_bits=window_bits  bin_pt=0  opselect=C  inp2=PCIN>>17  opr=+  inp1=P  carry=CIN  iostate=0  explicit_period=on  period=1  dbl_ovrd=off
  Constant3 : xbsIndex_r3/Constant  const=0  equ=P=C  arith_type=Unsigned  n_bits=sync_bits - x_int_bits - ant_bits - window_bits  bin_pt=0  opselect=C  inp2=PCIN>>17  opr=+  inp1=P  carry=CIN  iostate=0  explicit_period=on  period=1  dbl_ovrd=off
  Delay{1,4,6..7} (4 alike) : xbsIndex_r3/Delay  latency=1  reg_retiming=off  explicit_period=off  period=1  en=off  accept_only_valid=off  init_zero=on  dbl_ovrd=off  show_param=off
      settings: xl_area=[0, 0, 0, 0, 0, 0, 0]
  Gateway Out{1..6} (6 alike) : xbsIndex_r3/Gateway Out  output_type=Double  nbits=8  bin_pt=6  arith_type=Boolean  quantization=Truncate  overflow=Wrap  hdl_port=off  timing_constraint=None  locs_specified=off  LOCs={}  needs_fixed_name=off  show_param=off
      settings: xl_area=[0, 0, 0, 0, 0, 0, 0]
  Logical1 : xbsIndex_r3/Logical  logical_function=AND  inputs=2  precision=Full  arith_type=Unsigned  n_bits=8  bin_pt=2  align_bp=on  latency=0  explicit_period=off  period=1  en=off  dbl_ovrd=off  show_param=off
      settings: xl_area=[0, 0, 0, 0, 0, 0, 0]
  Logical2 : xbsIndex_r3/Logical  logical_function=AND  inputs=2  precision=Full  arith_type=Unsigned  n_bits=8  bin_pt=2  align_bp=on  latency=0  explicit_period=off  period=1  en=off  dbl_ovrd=off  show_param=off
      settings: xl_area=[0, 0, 0, 0, 0, 0, 0]
  Relational1 : xbsIndex_r3/Relational  mode=a>=b  latency=1  explicit_period=on  period=1  en=off  dbl_ovrd=off  show_param=off
      settings: xl_area=[0, 0, 0, 0, 0, 0, 0]
  Relational4 : xbsIndex_r3/Relational  mode=a=b  latency=1  explicit_period=off  period=1  en=off  dbl_ovrd=off  show_param=off
      settings: xl_area=[0, 0, 0, 0, 0, 0, 0]
  Slice1 : xbsIndex_r3/Slice  mode=Lower Bit Location + Width  nbits=window_bits  bit1=0  base1=MSB of Input  bit0=0  base0=LSB of Input  boolean_output=off  explicit_period=off  period=1  dbl_ovrd=off
  Slice2 : xbsIndex_r3/Slice  mode=Upper Bit Location + Width  nbits=1  bit1=0  base1=MSB of Input  bit0=0  base0=LSB of Input  boolean_output=on  explicit_period=off  period=1  dbl_ovrd=off
  Slice3 : xbsIndex_r3/Slice  mode=Lower Bit Location + Width  nbits=window_bits  bit1=0  base1=MSB of Input  bit0=0  base0=LSB of Input  boolean_output=off  explicit_period=off  period=1  dbl_ovrd=off
  Slice4 : xbsIndex_r3/Slice  mode=Lower Bit Location + Width  nbits=x_int_bits + ant_bits  bit1=0  base1=MSB of Input  bit0=0  base0=LSB of Input  boolean_output=off  explicit_period=off  period=1  dbl_ovrd=off
  Slice5 : xbsIndex_r3/Slice  mode=Two Bit Locations  nbits=window_bits  bit1=sync_bits - x_int_bits - ant_bits - 1  base1=LSB of Input  bit0=window_bits  base0=LSB of Input  boolean_output=off  explicit_period=off  period=1  dbl_ovrd=off
  Slice6 : xbsIndex_r3/Slice  mode=Upper Bit Location + Width  nbits=1  bit1=0  base1=MSB of Input  bit0=0  base0=LSB of Input  boolean_output=on  explicit_period=off  period=1  dbl_ovrd=off
  edge : casper_library/Misc/edge
  edge1 : casper_library/Misc/edge
  internal_descr_Scope : Scope  NumInputPorts=6
      settings: TimeRange=1  YMin=-1~-1~0.95~-5~-5~-5  YMax=1~1~1.05~5~5~5  SaveName=ScopeData2
  pulse_ext : casper_library/Misc/pulse_ext  pulse_len=2^(x_int_bits + ant_bits)
  win_addr_cnt : xbsIndex_r3/Counter  cnt_type=Free Running  n_bits=x_int_bits + ant_bits + 1  bin_pt=0  arith_type=Unsigned  start_count=0  cnt_to=Inf  cnt_by_val=1  operation=Up  explicit_period=off  period=1  load_pin=off  rst=off  en=off  dbl_ovrd=off  show_param=off  use_rpm=on  gen_core=off
      settings: xl_area=[0, 0, 0, 0, 0, 0, 0]
  win_cnt : xbsIndex_r3/Counter  cnt_type=Free Running  n_bits=window_bits + 1  bin_pt=0  arith_type=Unsigned  start_count=0  cnt_to=Inf  cnt_by_val=1  operation=Up  explicit_period=off  period=1  load_pin=off  rst=off  en=on  dbl_ovrd=off  show_param=off  use_rpm=on  gen_core=off
      settings: xl_area=[0, 0, 0, 0, 0, 0, 0]
  gen_sync : Outport
  rd_en : Outport  Port=2
  rd_addr : Outport  Port=3
  current_rd_window : Outport  Port=4
  wires:
  pulse_ext/1 -> Delay6/1
  Concat1/1 -> Delay4/1
  Delay7/1 -> Concat1/2
  Slice2/1 -> edge1/1
  Slice1/1 -> [current_window], Delay1/1
  Slice4/1 -> Delay7/1
  edge/1 -> Logical1/1
  Slice6/1 -> edge/1
  win_addr_cnt/1 -> Slice4/1, Slice6/1
  Slice5/1 -> Relational4/2
  Constant3/1 -> Relational4/1
  edge1/1 -> Logical2/1
  Logical1/1 -> pulse_ext/1, [ship_window_now]
  win_cnt/1 -> Slice2/1, Slice1/1
  maxcnt/1 -> Slice5/1, [maxcnt]
  Logical2/1 -> gen_sync/1
  Delay6/1 -> rd_en/1, Gateway Out1/1
  [ship_next_window] -> Logical1/2
  Delay4/1 -> rd_addr/1, Gateway Out2/1
  Slice3/1 -> AddSub1/1
  AddSub1/1 -> Relational1/1
  Constant1/1 -> Relational1/2
  [current_window] -> AddSub1/2
  [maxcnt] -> Slice3/1
  Relational1/1 -> [ship_next_window]
  [ship_window_now] -> win_cnt/1
  Relational4/1 -> Logical2/2
  Gateway Out3/1 -> internal_descr_Scope/2
  Gateway Out4/1 -> internal_descr_Scope/1
  Gateway Out5/1 -> internal_descr_Scope/3
  [maxcnt] -> Gateway Out4/1
  [current_window] -> Gateway Out3/1
  [ship_next_window] -> Gateway Out5/1
  [current_window] -> Concat1/1
  Gateway Out6/1 -> internal_descr_Scope/4
  Gateway Out1/1 -> internal_descr_Scope/5
  Gateway Out2/1 -> internal_descr_Scope/6
  [ship_window_now] -> Gateway Out6/1
  Delay1/1 -> current_rd_window/1

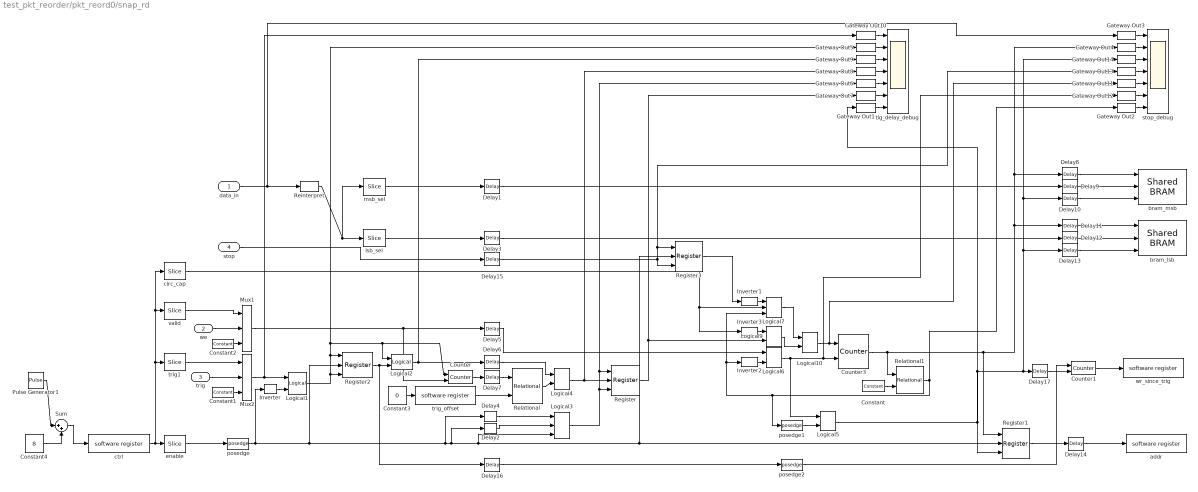
== system test_pkt_reorder/pkt_reord0/snap_rd ==
  data_in : Inport  Port=1  LatchInput=off
  we : Inport  Port=2  LatchInput=off
  trig : Inport  Port=3  LatchInput=off
  stop : Inport  Port=4  LatchInput=off
  Constant : xbsIndex_r3/Constant  const=(2^nsamples)-1  equ=P=C  arith_type=Unsigned  n_bits=nsamples  bin_pt=0  opselect=C  inp2=PCIN>>17  opr=+  inp1=P  carry=CIN  iostate=0  explicit_period=off  period=1  dbl_ovrd=off
  Constant1 : xbsIndex_r3/Constant  const=1  equ=P=C  arith_type=Boolean  n_bits=1  bin_pt=0  opselect=C  inp2=PCIN>>17  opr=+  inp1=P  carry=CIN  iostate=0  explicit_period=on  period=1  dbl_ovrd=off
  Constant2 : xbsIndex_r3/Constant  const=1  equ=P=C  arith_type=Boolean  n_bits=1  bin_pt=0  opselect=C  inp2=PCIN>>17  opr=+  inp1=P  carry=CIN  iostate=0  explicit_period=on  period=1  dbl_ovrd=off
  Constant3 : Constant  Value=0
  Constant4 : Constant  Value=8
  Counter : xbsIndex_r3/Counter  cnt_type=Free Running  n_bits=32  bin_pt=0  arith_type=Unsigned  start_count=1  cnt_to=Inf  cnt_by_val=1  operation=Up  explicit_period=on  period=1  load_pin=off  rst=on  en=on  dbl_ovrd=off  show_param=off  use_rpm=on  gen_core=off
      settings: xl_area=[0, 0, 0, 0, 0, 0, 0]
  Counter1 : xbsIndex_r3/Counter  cnt_type=Free Running  n_bits=32  bin_pt=0  arith_type=Unsigned  start_count=1  cnt_to=Inf  cnt_by_val=1  operation=Up  explicit_period=on  period=1  load_pin=off  rst=on  en=on  dbl_ovrd=off  show_param=off  use_rpm=on  gen_core=off
      settings: xl_area=[0, 0, 0, 0, 0, 0, 0]
  Counter3 : xbsIndex_r3/Counter  cnt_type=Count Limited  n_bits=nsamples  bin_pt=0  arith_type=Unsigned  start_count=0  cnt_to=(2^nsamples)-1  cnt_by_val=1  operation=Up  explicit_period=on  period=1  load_pin=off  rst=on  en=on  dbl_ovrd=off  show_param=off  use_rpm=on  gen_core=off
      settings: xl_area=[0, 0, 0, 0, 0, 0, 0]
  Delay{1,3..7,15..16} (8 alike) : xbsIndex_r3/Delay  latency=1  reg_retiming=on  explicit_period=on  period=1  en=off  accept_only_valid=off  init_zero=on  dbl_ovrd=off  show_param=off
      settings: xl_area=[0, 0, 0, 0, 0, 0, 0]
  Delay{2,8..14,17} (9 alike) : xbsIndex_r3/Delay  latency=2  reg_retiming=on  explicit_period=on  period=1  en=off  accept_only_valid=off  init_zero=on  dbl_ovrd=off  show_param=off
      settings: xl_area=[0, 0, 0, 0, 0, 0, 0]
  Gateway Out{1..14} (14 alike) : xbsIndex_r3/Gateway Out  output_type=Double  nbits=8  bin_pt=6  arith_type=Boolean  quantization=Truncate  overflow=Wrap  hdl_port=off  timing_constraint=None  locs_specified=off  LOCs={}  needs_fixed_name=off  show_param=off
      settings: xl_area=[0, 0, 0, 0, 0, 0, 0]
  Inverter{,1..3} (4 alike) : xbsIndex_r3/Inverter  latency=0  explicit_period=off  period=1  en=off  dbl_ovrd=off  show_param=off
      settings: xl_area=[0, 0, 0, 0, 0, 0, 0]
  Logical1 : xbsIndex_r3/Logical  logical_function=AND  inputs=2  precision=Full  arith_type=Unsigned  n_bits=8  bin_pt=2  align_bp=on  latency=0  explicit_period=off  period=1  en=off  dbl_ovrd=off  show_param=off
      settings: xl_area=[0, 0, 0, 0, 0, 0, 0]
  Logical10 : xbsIndex_r3/Logical  logical_function=OR  inputs=2  precision=Full  arith_type=Unsigned  n_bits=8  bin_pt=2  align_bp=on  latency=0  explicit_period=off  period=1  en=off  dbl_ovrd=off  show_param=off
      settings: xl_area=[0, 0, 0, 0, 0, 0, 0]
  Logical2 : xbsIndex_r3/Logical  logical_function=OR  inputs=2  precision=Full  arith_type=Unsigned  n_bits=8  bin_pt=2  align_bp=on  latency=0  explicit_period=on  period=1  en=off  dbl_ovrd=off  show_param=off
      settings: xl_area=[0, 0, 0, 0, 0, 0, 0]
  Logical3 : xbsIndex_r3/Logical  logical_function=OR  inputs=3  precision=Full  arith_type=Unsigned  n_bits=8  bin_pt=2  align_bp=on  latency=0  explicit_period=on  period=1  en=off  dbl_ovrd=off  show_param=off
      settings: xl_area=[0, 0, 0, 0, 0, 0, 0]
  Logical4 : xbsIndex_r3/Logical  logical_function=AND  inputs=2  precision=Full  arith_type=Unsigned  n_bits=8  bin_pt=2  align_bp=on  latency=0  explicit_period=on  period=1  en=off  dbl_ovrd=off  show_param=off
      settings: xl_area=[0, 0, 0, 0, 0, 0, 0]
  Logical5 : xbsIndex_r3/Logical  logical_function=OR  inputs=2  precision=Full  arith_type=Unsigned  n_bits=8  bin_pt=2  align_bp=on  latency=0  explicit_period=off  period=1  en=off  dbl_ovrd=off  show_param=off
      settings: xl_area=[0, 0, 0, 0, 0, 0, 0]
  Logical6 : xbsIndex_r3/Logical  logical_function=AND  inputs=2  precision=Full  arith_type=Unsigned  n_bits=8  bin_pt=2  align_bp=on  latency=0  explicit_period=off  period=1  en=off  dbl_ovrd=off  show_param=off
      settings: xl_area=[0, 0, 0, 0, 0, 0, 0]
  Logical7 : xbsIndex_r3/Logical  logical_function=AND  inputs=3  precision=Full  arith_type=Unsigned  n_bits=8  bin_pt=2  align_bp=on  latency=0  explicit_period=off  period=1  en=off  dbl_ovrd=off  show_param=off
      settings: xl_area=[0, 0, 0, 0, 0, 0, 0]
  Logical9 : xbsIndex_r3/Logical  logical_function=AND  inputs=2  precision=Full  arith_type=Unsigned  n_bits=8  bin_pt=2  align_bp=on  latency=0  explicit_period=off  period=1  en=off  dbl_ovrd=off  show_param=off
      settings: xl_area=[0, 0, 0, 0, 0, 0, 0]
  Mux1 : xbsIndex_r3/Mux  inputs=2  precision=Full  arith_type="Signed  (2's comp)"  n_bits=8  bin_pt=2  quantization=Truncate  overflow=Wrap  latency=0  explicit_period=off  period=1  en=off  dbl_ovrd=off  show_param=off  mux_type=off  use_rpm=off  gen_core=off
      settings: xl_area=[0, 0, 0, 0, 0, 0, 0]
  Mux2 : xbsIndex_r3/Mux  inputs=2  precision=Full  arith_type="Signed  (2's comp)"  n_bits=8  bin_pt=2  quantization=Truncate  overflow=Wrap  latency=0  explicit_period=off  period=1  en=off  dbl_ovrd=off  show_param=off  mux_type=off  use_rpm=off  gen_core=off
      settings: xl_area=[0, 0, 0, 0, 0, 0, 0]
  Pulse Generator1 : DiscretePulseGenerator  Period=4196  PulseWidth=2
  Register{,1..3} (4 alike) : xbsIndex_r3/Register  init=0  reg_only_valid=off  explicit_period=off  period=1  rst=on  en=on  out_en=off  dbl_ovrd=off  show_param=off
      settings: xl_area=[0, 0, 0, 0, 0, 0, 0]
  Reinterpret : xbsIndex_r3/Reinterpret  force_arith_type=on  arith_type=Unsigned  force_bin_pt=on  bin_pt=0  force_valid=on
  Relational : xbsIndex_r3/Relational  mode=a>=b  latency=0  explicit_period=on  period=1  en=off  dbl_ovrd=off  show_param=off
      settings: xl_area=[0, 0, 0, 0, 0, 0, 0]
  Relational1 : xbsIndex_r3/Relational  mode=a=b  latency=0  explicit_period=off  period=1  en=off  dbl_ovrd=off  show_param=off
      settings: xl_area=[0, 0, 0, 0, 0, 0, 0]
  Sum : Sum  Inputs=|++
  addr : xps_library/software register  Tag=xps:sw_reg  io_dir=To Processor  arith_type=Unsigned  bitwidth=32  bin_pt=0  sample_period=1  gw_name=b_2x_8a_r310a_reord0_snap_rd_addr_user_data_in
  bram_lsb : xps_library/Shared BRAM  Tag=xps:bram  arith_type=Unsigned  addr_width=nsamples  data_width=32  data_bin_pt=0  init_vals=0  sample_rate=1
  bram_msb : xps_library/Shared BRAM  Tag=xps:bram  arith_type=Unsigned  addr_width=nsamples  data_width=32  data_bin_pt=0  init_vals=0  sample_rate=1
  circ_cap : xbsIndex_r3/Slice  mode=Lower Bit Location + Width  nbits=1  bit1=0  base1=LSB of Input  bit0=3  base0=LSB of Input  boolean_output=on  explicit_period=off  period=1  dbl_ovrd=off
  ctrl : xps_library/software register  Tag=xps:sw_reg  io_dir=From Processor  arith_type=Unsigned  bitwidth=32  bin_pt=0  sample_period=1  gw_name=b_2x_8a_r310a_reord0_snap_rd_ctrl_user_data_out
  enable : xbsIndex_r3/Slice  mode=Lower Bit Location + Width  nbits=1  bit1=0  base1=LSB of Input  bit0=0  base0=LSB of Input  boolean_output=on  explicit_period=on  period=1  dbl_ovrd=off
  lsb_sel : xbsIndex_r3/Slice  mode=Lower Bit Location + Width  nbits=32  bit1=0  base1=LSB of Input  bit0=0  base0=LSB of Input  boolean_output=on  explicit_period=on  period=1  dbl_ovrd=off
  msb_sel : xbsIndex_r3/Slice  mode=Lower Bit Location + Width  nbits=32  bit1=0  base1=LSB of Input  bit0=32  base0=LSB of Input  boolean_output=on  explicit_period=on  period=1  dbl_ovrd=off
  posedge : casper_library/Misc/posedge  Tag=Rising Edge Detector
  posedge1 : casper_library/Misc/posedge  Tag=Rising Edge Detector
  posedge2 : casper_library/Misc/posedge  Tag=Rising Edge Detector
  stop_debug : Scope  NumInputPorts=7
      settings: YMin=272014000~0~0~-5~-5~-5~-5  YMax=300648000~110~1~5~5~5~5  SaveName=ScopeData4
  tig_delay_debug : Scope  NumInputPorts=7
      settings: YMin=2.72014e+008~0~0~-5~-5~-5~-5  YMax=3.00648e+008~110~1~5~5~5~5  SaveName=ScopeData3
  trig1 : xbsIndex_r3/Slice  mode=Lower Bit Location + Width  nbits=1  bit1=0  base1=LSB of Input  bit0=1  base0=LSB of Input  boolean_output=on  explicit_period=off  period=1  dbl_ovrd=off
  trig_offset : xps_library/software register  Tag=xps:sw_reg  io_dir=From Processor  arith_type=Unsigned  bitwidth=32  bin_pt=0  sample_period=1  gw_name=b_2x_8a_r310a_reord0_snap_rd_trig_offset_user_data_out
  valid : xbsIndex_r3/Slice  mode=Lower Bit Location + Width  nbits=1  bit1=0  base1=LSB of Input  bit0=2  base0=LSB of Input  boolean_output=on  explicit_period=off  period=1  dbl_ovrd=off
  wr_since_trig : xps_library/software register  Tag=xps:sw_reg  io_dir=To Processor  arith_type=Unsigned  bitwidth=32  bin_pt=0  sample_period=1  gw_name=b_2x_8a_r310a_reord0_snap_rd_wr_since_trig_user_data_in
  wires:
  data_in/1 -> Reinterpret/1, Gateway Out3/1
  Register/1 -> Gateway Out7/1, Logical9/2
  Mux2/1 -> Logical1/1, Gateway Out10/1
  Inverter/1 -> Logical1/2
  valid/1 -> Mux1/1
  trig1/1 -> Mux2/1
  Register1/1 -> Delay14/1
  Constant2/1 -> Mux1/3
  we/1 -> Mux1/2
  Mux1/1 -> Delay5/1, Counter/2
  Constant1/1 -> Mux2/3
  posedge/1 -> Inverter/1, Register2/2, Delay4/1, Logical3/3, Register3/2, Register1/2, Delay2/1
  ctrl/1 -> trig1/1, valid/1, circ_cap/1, enable/1
  enable/1 -> posedge/1
  trig/1 -> Mux2/2
  Logical4/1 -> Register/2, Gateway Out8/1
  Logical1/1 -> Register2/1, Logical2/1, Counter/1, Gateway Out5/1, Register2/3
  Register2/1 -> Logical2/2, Delay16/1
  Delay4/1 -> Logical3/1
  Logical3/1 -> Register/3, Register/1, Gateway Out6/1
  Constant3/1 -> trig_offset/1
  trig_offset/1 -> Relational/2
  Relational/1 -> Logical4/2
  Logical2/1 -> Gateway Out9/1, Delay6/1
  Counter/1 -> Delay7/1
  Delay2/1 -> Logical3/2
  Delay5/1 -> Logical6/1
  Delay6/1 -> Logical4/1
  Delay7/1 -> Relational/1
  Gateway Out9/1 -> tig_delay_debug/3
  Gateway Out5/1 -> tig_delay_debug/2
  Gateway Out8/1 -> tig_delay_debug/4
  Gateway Out6/1 -> tig_delay_debug/5
  Gateway Out10/1 -> tig_delay_debug/1
  Gateway Out7/1 -> tig_delay_debug/6
  Gateway Out1/1 -> tig_delay_debug/7
  Reinterpret/1 -> lsb_sel/1, msb_sel/1
  lsb_sel/1 -> Delay3/1
  msb_sel/1 -> Delay1/1
  Delay1/1 -> Delay9/1
  Delay3/1 -> Delay12/1
  Delay8/1 -> bram_msb/1
  Delay9/1 -> bram_msb/2
  Delay10/1 -> bram_msb/3
  Delay11/1 -> bram_lsb/1
  Delay12/1 -> bram_lsb/2
  Delay13/1 -> bram_lsb/3
  Delay14/1 -> addr/1
  Logical6/1 -> Counter3/2, Gateway Out12/1, Logical5/1
  Counter3/1 -> Register1/1, Delay8/1, Gateway Out4/1, Delay11/1, Relational1/1
  Constant/1 -> Relational1/2
  Relational1/1 -> Gateway Out2/1, Inverter2/1, Logical7/3, posedge1/1
  circ_cap/1 -> Logical7/2, Inverter3/1
  stop/1 -> Delay15/1
  Register3/1 -> Inverter1/1
  Delay15/1 -> Register3/3, Register3/1, Gateway Out13/1
  Inverter1/1 -> Logical7/1
  Logical7/1 -> Logical10/1
  Logical10/1 -> Counter3/1, Gateway Out11/1
  Inverter3/1 -> Logical9/1
  Logical9/1 -> Logical10/2
  Gateway Out14/1 -> stop_debug/3
  Gateway Out4/1 -> stop_debug/2
  Gateway Out13/1 -> stop_debug/4
  Gateway Out11/1 -> stop_debug/5
  Gateway Out3/1 -> stop_debug/1
  Gateway Out12/1 -> stop_debug/6
  Gateway Out2/1 -> stop_debug/7
  Inverter2/1 -> Logical6/2
  Constant4/1 -> Sum/2
  Sum/1 -> ctrl/1
  Pulse Generator1/1 -> Sum/1
  Logical5/1 -> Register1/3, Gateway Out14/1, Delay10/1, Delay13/1, Delay17/1, Gateway Out1/1
  posedge1/1 -> Logical5/2
  Counter1/1 -> wr_since_trig/1
  posedge2/1 -> Counter1/1
  Delay16/1 -> posedge2/1
  Delay17/1 -> Counter1/2
